simulink model "controladorPaola22a"  (R2022a)
settings: Solver=ode23t  StartTime=0.0  StopTime=60  MaxStep=1e-3  RelTol=1e-3
values from neighbouring files (symbols this model uses):
  AL = double(subs(A_par))    [ANTImodeloMATEMATICOFINAL.m]
  BL = double(subs(B_par))    [ANTImodeloMATEMATICOFINAL.m]
  Blo = 8.18575752786119e-06    (= 8.18575752786e-06)    [ANTImodeloMATEMATICOFINAL.m]
  Bmo = 2.02156082362446e-07    (= 2.02156082362e-07)    [ANTImodeloMATEMATICOFINAL.m]
  CL = double(subs(C_par))    [ANTImodeloMATEMATICOFINAL.m]
  DL = double(subs(D_par))    [ANTImodeloMATEMATICOFINAL.m]
  do = 0.06862-0.021    (= 0.04762)    [ANTImodeloMATEMATICOFINAL.m]
  go = 9.81    [ANTImodeloMATEMATICOFINAL.m]
  Jlo = 0.00100697016255642    (= 0.00100697016256)    [ANTImodeloMATEMATICOFINAL.m]
  Jmo = 2.08549279330578e-07    (= 2.08549279331e-07)    [ANTImodeloMATEMATICOFINAL.m]
  Kes = K(:,1:n)    [ANTImodeloMATEMATICOFINAL.m]
  Ki = -K(:,n+1:end)    [ANTImodeloMATEMATICOFINAL.m]
  Kio = 0.00119530882984502    (= 0.00119530882985)    [ANTImodeloMATEMATICOFINAL.m]
  Kvo = 0.0035694528924319    (= 0.00356945289243)    [ANTImodeloMATEMATICOFINAL.m]
  Lo = 0.667669785204658    (= 0.667669785205)    [ANTImodeloMATEMATICOFINAL.m]
  mo = 0.17244    [ANTImodeloMATEMATICOFINAL.m]
  no = 120    [ANTImodeloMATEMATICOFINAL.m]
  Ro = 5.15610211779038    (= 5.15610211779)    [ANTImodeloMATEMATICOFINAL.m]
  Vin0 = Ro*X10    (= 0)    [ANTImodeloMATEMATICOFINAL.m]
  X10 = 0    [ANTImodeloMATEMATICOFINAL.m]
  X20 = 0    [ANTImodeloMATEMATICOFINAL.m]
settings Model: Creator=hubertdelgado  LastModifiedBy=electronica
settings DebuggingCC: UnconnectedInputMsg=warning  UnconnectedOutputMsg=warning  UnconnectedLineMsg=warning
settings RTWCC: DLArmComputeVersion=19.05

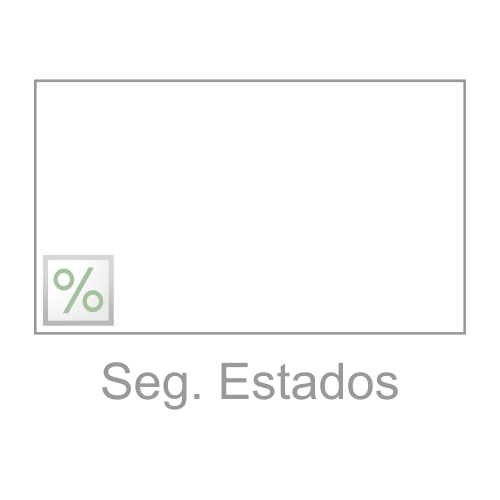
[thumbnail: Simulink's stored preview of the top-level diagram]
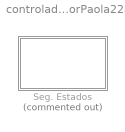
== system controladorPaola22a ==
  Seg. Estados : Subsystem  Commented=on

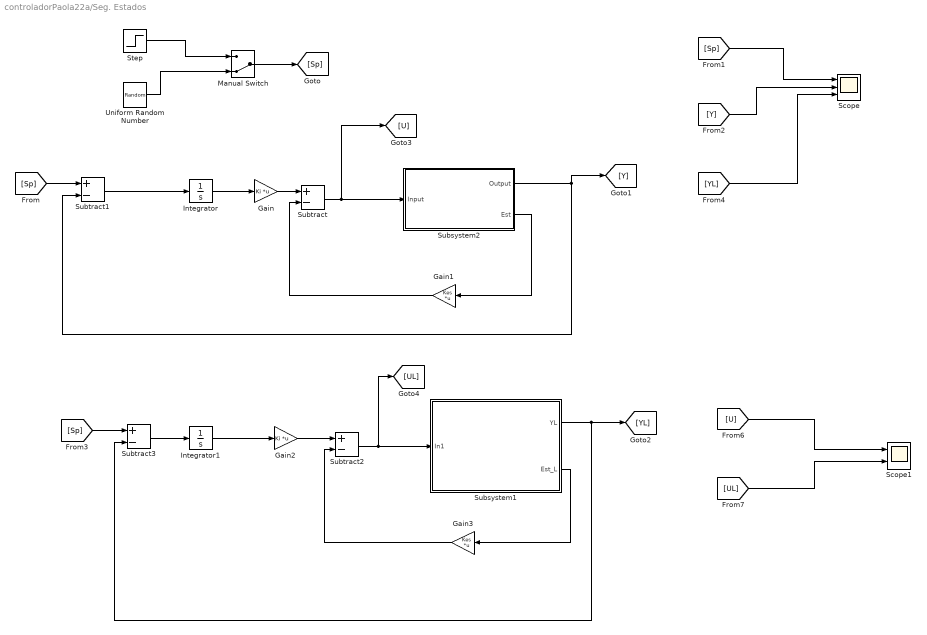
== system controladorPaola22a/Seg. Estados ==
  Gain : Gain  Gain=Ki  Multiplication=Matrix(K*u)
  Gain1 : Gain  Gain=Kes  Multiplication=Matrix(K*u)
  Gain2 : Gain  Gain=Ki  Multiplication=Matrix(K*u)
  Gain3 : Gain  Gain=Kes  Multiplication=Matrix(K*u)
  Integrator : Integrator
  Integrator1 : Integrator
  Manual Switch : ManualSwitch  CurrentSetting=0
  Scope : Scope  NumInputPorts=3
  Scope1 : Scope  NumInputPorts=2
  Step : Step  Time=0  After=0  SampleTime=0
  Subsystem1 : Subsystem
  Subsystem2 : Subsystem
  Subtract{,1..3} (4 alike) : Sum  Inputs=+-
  Uniform Random Number : UniformRandomNumber  Minimum=-120*(pi/180)  Maximum=120*(pi/180)  SampleTime=10
  wires:
  Subsystem2/1(Output) -> Subtract1/2, [Y]
  Subsystem2/2(Est) -> Gain1/1
  Subtract/1 -> Subsystem2/1(Input), [U]
  Gain1/1 -> Subtract/2
  Subtract2/1 -> [UL], Subsystem1/1(In1)
  Gain/1 -> Subtract/1
  [Sp] -> Subtract1/1
  [Sp] -> Subtract3/1
  Gain2/1 -> Subtract2/1
  Subsystem1/1(YL) -> [YL], Subtract3/2
  Subsystem1/2(Est_L) -> Gain3/1
  Gain3/1 -> Subtract2/2
  Integrator/1 -> Gain/1
  Subtract1/1 -> Integrator/1
  Integrator1/1 -> Gain2/1
  Subtract3/1 -> Integrator1/1
  [UL] -> Scope1/2
  Step/1 -> Manual Switch/1
  Manual Switch/1 -> [Sp]
  [Y] -> Scope/2
  [Sp] -> Scope/1
  [YL] -> Scope/3
  [U] -> Scope1/1
  Uniform Random Number/1 -> Manual Switch/2

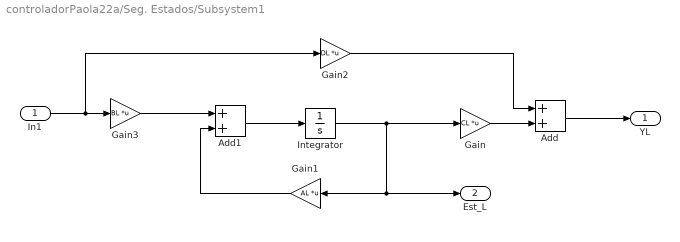
== system controladorPaola22a/Seg. Estados/Subsystem1 ==
  In1 : Inport
  Add : Sum
  Add1 : Sum
  Gain : Gain  Gain=CL  Multiplication=Matrix(K*u)
  Gain1 : Gain  Gain=AL  Multiplication=Matrix(K*u)
  Gain2 : Gain  Gain=DL  Multiplication=Matrix(K*u)
  Gain3 : Gain  Gain=BL  Multiplication=Matrix(K*u)
  Integrator : Integrator
  YL : Outport
  Est_L : Outport  Port=2
  wires:
  Gain/1 -> Add/2
  Integrator/1 -> Gain/1, Est_L/1, Gain1/1
  Add1/1 -> Integrator/1
  Gain1/1 -> Add1/2
  Gain2/1 -> Add/1
  Gain3/1 -> Add1/1
  Add/1 -> YL/1
  In1/1 -> Gain2/1, Gain3/1

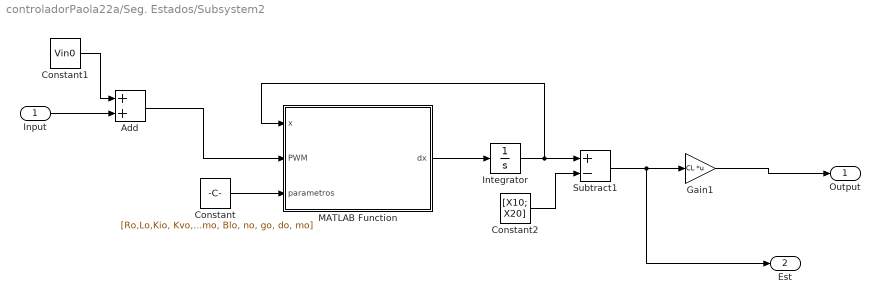
== system controladorPaola22a/Seg. Estados/Subsystem2 ==
  Input : Inport
  Add : Sum
  Constant : Constant  Value=[Ro,Lo,Kio, Kvo, Jmo, Jlo, Bmo, Blo, no, go, do, mo]
  Constant1 : Constant  Value=Vin0
  Constant2 : Constant  Value=[X10; X20]
  Gain1 : Gain  Gain=CL  Multiplication=Matrix(K*u)
  Integrator : Integrator  InitialCondition=[X10; X20]
  MATLAB Function : MATLAB Function  TreatAsAtomicUnit=on
  Subtract1 : Sum  Inputs=+-
  Output : Outport
  Est : Outport  Port=2
  wires:
  Add/1 -> MATLAB Function/2(PWM)
  Constant2/1 -> Subtract1/2
  Constant1/1 -> Add/1
  Input/1 -> Add/2
  MATLAB Function/1(dx) -> Integrator/1
  Constant/1 -> MATLAB Function/3(parametros)
  Integrator/1 -> Subtract1/1, MATLAB Function/1(x)
  Subtract1/1 -> Est/1, Gain1/1
  Gain1/1 -> Output/1

== matlab function controladorPaola22a/Seg. Estados/Subsystem2/MATLAB Function ==
  data: x input; PWM input; dx output; parametros input
function dx = fcn(x,PWM,parametros)

%ESTADOS
x1 = x(1);
x2 = x(2);

%Parametros
R = parametros(1);
L = parametros(2);
Ki = parametros(3);
Kv = parametros(4);
Jm = parametros(5);
Jl = parametros(6);
Bm = parametros(7);
Bl = parametros(8);
n = parametros(9);
g = parametros(10);
d = parametros(11);
m = parametros(12);

%EXPRESIONES
f1 = x2; %d0l/dt = Wl
f2= ((Ki*(((7*PWM/100)-(Kv*x2*n)/R))*n)-x2*(Bm*n^2+Bl)-(m*g*d*sin(x1)))/(Jl+Jm*n^2);

dx = [f1; f2];
